simulink model "test1"  (R2024a)
settings: Solver=FixedStepAuto  StartTime=0.0  StopTime=0.5  RelTol=1e-3
settings Model: Creator=hp  LastModifiedBy=Dell

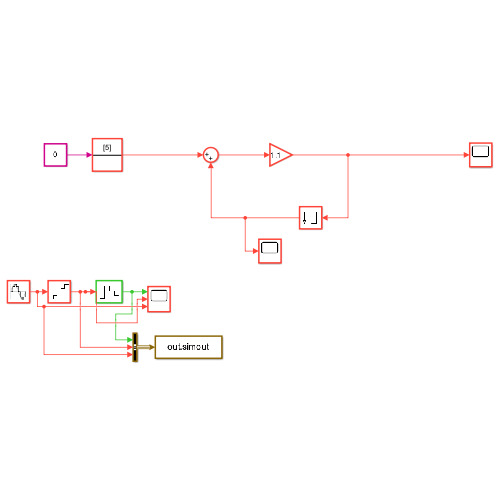
[thumbnail: Simulink's stored preview of the top-level diagram]
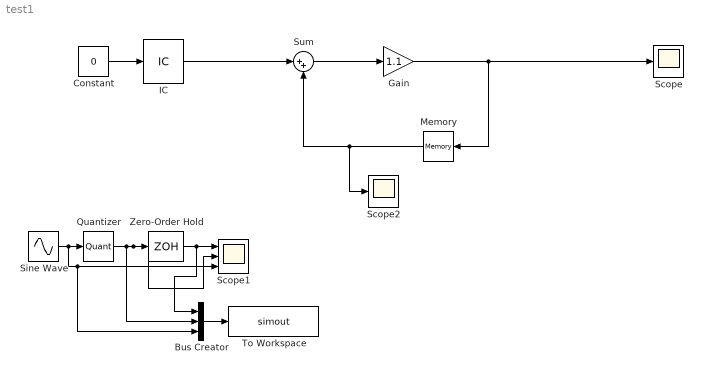
== system test1 ==
  Bus Creator : BusCreator  Inputs=3
  Constant : Constant  Value=0
  Gain : Gain  Gain=1.1
  IC : InitialCondition  Value=5
  Memory : Memory
  Quantizer : Quantizer  QuantizationInterval=0.1
  Scope : Scope
  Scope1 : Scope  NumInputPorts=3
  Scope2 : Scope
  Sine Wave : Sin  SampleTime=0.1
  Sum : Sum  Inputs=|++
  To Workspace : ToWorkspace  VariableName=simout  SaveFormat=Timeseries  SampleTime=-1
  Zero-Order Hold : ZeroOrderHold  SampleTime=0.5
  wires:
  Sine Wave/1 -> Bus Creator/3, Scope1/3, Quantizer/1
  Zero-Order Hold/1 -> Bus Creator/1, Scope1/1
  Quantizer/1 -> Bus Creator/2, Scope1/2, Zero-Order Hold/1
  Bus Creator/1 -> To Workspace/1
  Constant/1 -> IC/1
  IC/1 -> Sum/1
  Memory/1 -> Scope2/1, Sum/2
  Sum/1 -> Gain/1
  Gain/1 -> Memory/1, Scope/1
